simulink model "lab4"  (R2021a)
settings: Solver=VariableStepAuto  StartTime=0.0  StopTime=10.0  MaxStep=1e-3  RelTol=1e-3
libraries: simulink x7
settings Model: Creator=reemb  LastModifiedBy=reemb

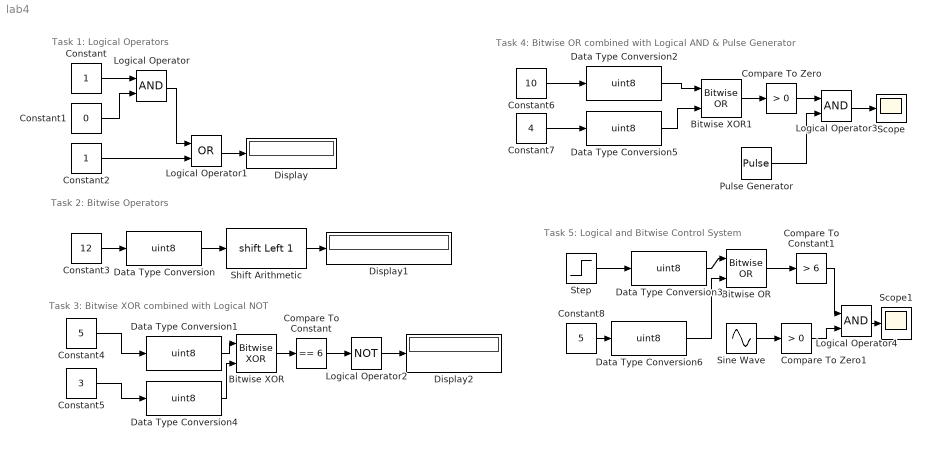
== system lab4 ==
  note: Task 5: Logical and Bitwise Control System
  note: Task 4: Bitwise OR combined with Logical AND & Pulse Generator
  note: Task 3: Bitwise XOR combined with Logical NOT
  note: Task 2: Bitwise Operators
  note: Task 1: Logical Operators
  Bitwise OR : simulink/Logic and Bit Operations/Bitwise Operator  logicop=OR  UseBitMask=off  NumInputPorts=2  BitMask=bin2dec('11011001')  BitMaskRealWorld=Stored Integer
  Bitwise XOR : simulink/Logic and Bit Operations/Bitwise Operator  logicop=XOR  UseBitMask=off  NumInputPorts=2  BitMask=bin2dec('11011001')  BitMaskRealWorld=Stored Integer
  Bitwise XOR1 : simulink/Logic and Bit Operations/Bitwise Operator  logicop=OR  UseBitMask=off  NumInputPorts=2  BitMask=bin2dec('11011001')  BitMaskRealWorld=Stored Integer
  Compare To Constant : simulink/Logic and Bit Operations/Compare To Constant  relop===  const=6  OutDataTypeStr=boolean
  Compare To Constant1 : simulink/Logic and Bit Operations/Compare To Constant  relop=>  const=6  OutDataTypeStr=boolean
  Compare To Zero : simulink/Logic and Bit Operations/Compare To Zero  relop=>  OutDataTypeStr=boolean
  Compare To Zero1 : simulink/Logic and Bit Operations/Compare To Zero  relop=>  OutDataTypeStr=boolean
  Constant : Constant
  Constant1 : Constant  Value=0
  Constant2 : Constant
  Constant3 : Constant  Value=12
  Constant4 : Constant  Value=5
  Constant5 : Constant  Value=3
  Constant6 : Constant  Value=10
  Constant7 : Constant  Value=4
  Constant8 : Constant  Value=5
  Data Type Conversion{,1..2,4..5} (5 alike) : DataTypeConversion  OutDataTypeStr=uint8  RndMeth=Round
  Data Type Conversion3 : DataTypeConversion  OutDataTypeStr=uint8
  Data Type Conversion6 : DataTypeConversion  OutDataTypeStr=uint8
  Display : Display
  Display1 : Display
  Display2 : Display
  Logical Operator : Logic  AllPortsSameDT=off  OutDataTypeStr=boolean
  Logical Operator1 : Logic  Operator=OR  AllPortsSameDT=off  OutDataTypeStr=boolean
  Logical Operator2 : Logic  Operator=NOT  AllPortsSameDT=off  OutDataTypeStr=boolean
  Logical Operator3 : Logic  AllPortsSameDT=off  OutDataTypeStr=boolean
  Logical Operator4 : Logic  AllPortsSameDT=off  OutDataTypeStr=boolean
  Pulse Generator : DiscretePulseGenerator  PulseType=Time based  PulseWidth=50
  Scope : Scope
  Scope1 : Scope
  Shift Arithmetic : ArithShift  BitShiftNumber=1  BitShiftDirection=Left
  Sine Wave : Sin  SampleTime=0
  Step : Step  Time=5  After=3  SampleTime=0
  wires:
  Constant/1 -> Logical Operator/1
  Constant1/1 -> Logical Operator/2
  Logical Operator/1 -> Logical Operator1/1
  Constant2/1 -> Logical Operator1/2
  Logical Operator1/1 -> Display/1
  Constant3/1 -> Data Type Conversion/1
  Shift Arithmetic/1 -> Display1/1
  Data Type Conversion/1 -> Shift Arithmetic/1
  Constant5/1 -> Data Type Conversion4/1
  Bitwise XOR/1 -> Compare To Constant/1
  Data Type Conversion1/1 -> Bitwise XOR/1
  Compare To Constant/1 -> Logical Operator2/1
  Logical Operator2/1 -> Display2/1
  Constant4/1 -> Data Type Conversion1/1
  Constant6/1 -> Data Type Conversion2/1
  Constant7/1 -> Data Type Conversion5/1
  Bitwise XOR1/1 -> Compare To Zero/1
  Data Type Conversion2/1 -> Bitwise XOR1/1
  Compare To Zero/1 -> Logical Operator3/1
  Pulse Generator/1 -> Logical Operator3/2
  Logical Operator3/1 -> Scope/1
  Step/1 -> Data Type Conversion3/1
  Data Type Conversion3/1 -> Bitwise OR/1
  Bitwise OR/1 -> Compare To Constant1/1
  Sine Wave/1 -> Compare To Zero1/1
  Compare To Zero1/1 -> Logical Operator4/2
  Compare To Constant1/1 -> Logical Operator4/1
  Logical Operator4/1 -> Scope1/1
  Data Type Conversion4/1 -> Bitwise XOR/2
  Data Type Conversion5/1 -> Bitwise XOR1/2
  Constant8/1 -> Data Type Conversion6/1
  Data Type Conversion6/1 -> Bitwise OR/2
